simulink model "UnbalancedStarConnectedLoad1"  (Simulink 10.3)
settings: Solver=ode45  StartTime=0.0  StopTime=0.1  RelTol=1e-3  EnableMultiTasking=on
libraries: spsSeriesRLCBranchLib x5, spsACVoltageSourceLib x3, spsVoltageMeasurementLib x3, spsThreePhaseVIMeasurementLib x1, spsCurrentMeasurementLib x1, spspowerguiLib x1
settings Model: Creator=bas  LastModifiedBy=Rahul
settings DataIOCC: LimitDataPoints=on
settings DebuggingCC: SolverPrmCheckMsg=warning

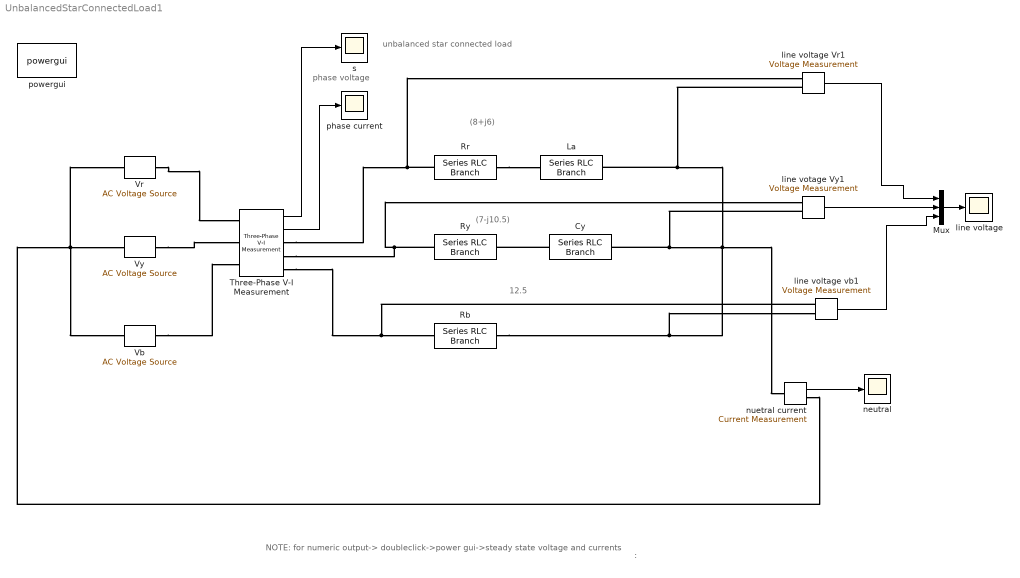
== system UnbalancedStarConnectedLoad1 ==
  note: (8+j6)
  note: (7-j10.5)
  note: 12.5
  note: :
  note: NOTE: for numeric output-> doubleclick->power gui->steady state voltage and currents
  note: unbalanced star connected load
  note: phase voltage
  " Cy" : spsSeriesRLCBranchLib/Series RLC Branch  LConnTagsString=__new0  RConnTagsString=__new0  BranchType=C  Resistance=7  Inductance=1e-3  SetiL0=off  InitialCurrent=0  Capacitance=303.15e-6  Setx0=off  InitialVoltage=0  Measurements=None
  " Ry" : spsSeriesRLCBranchLib/Series RLC Branch  LConnTagsString=__new0  RConnTagsString=__new0  BranchType=R  Resistance=7  Inductance=1e-3  SetiL0=off  InitialCurrent=0  Capacitance=1e-6  Setx0=off  InitialVoltage=0  Measurements=None
  La : spsSeriesRLCBranchLib/Series RLC Branch  LConnTagsString=__new0  RConnTagsString=__new0  BranchType=L  Resistance=15  Inductance=0.019  SetiL0=off  InitialCurrent=0  Capacitance=1e-6  Setx0=off  InitialVoltage=0  Measurements=None
  Mux : Mux  Inputs=3
  Rb : spsSeriesRLCBranchLib/Series RLC Branch  LConnTagsString=__new0  RConnTagsString=__new0  BranchType=R  Resistance=12.5  Inductance=1e-3  SetiL0=off  InitialCurrent=0  Capacitance=1e-6  Setx0=off  InitialVoltage=0  Measurements=None
  Rr : spsSeriesRLCBranchLib/Series RLC Branch  LConnTagsString=__new0  RConnTagsString=__new0  BranchType=R  Resistance=8  Inductance=1e-3  SetiL0=off  InitialCurrent=0  Capacitance=1e-6  Setx0=off  InitialVoltage=0  Measurements=None
  Three-Phase V-I Measurement : spsThreePhaseVIMeasurementLib/Three-Phase V-I Measurement  VoltageMeasurement=phase-to-phase  SetLabelV=off  LabelV=Vabc  Vpu=off  VpuLL=off  CurrentMeasurement=yes  SetLabelI=off  LabelI=Iabc  Ipu=off  Pbase=100e6  Vbase=500e3  OutputType=Complex  PhasorSimulation=off  PSBequivalent=0
  Vb : spsACVoltageSourceLib/AC Voltage Source  Amplitude=254  Phase=120  Frequency=50  SampleTime=0  Measurements=None  BusType=swing  Pref=10e3  Qref=0  Qmin=-inf  Qmax=+inf
  Vr : spsACVoltageSourceLib/AC Voltage Source  Amplitude=254  Phase=0  Frequency=50  SampleTime=0  Measurements=None  BusType=swing  Pref=10e3  Qref=0  Qmin=-inf  Qmax=+inf
  Vy : spsACVoltageSourceLib/AC Voltage Source  Amplitude=254  Phase=-120  Frequency=50  SampleTime=0  Measurements=None  BusType=swing  Pref=10e3  Qref=0  Qmin=-inf  Qmax=+inf
  line voltage : Scope
  line voltage Vr1 : spsVoltageMeasurementLib/Voltage Measurement  PhasorSimulation=off  OutputType=Complex  PSBequivalent=0
  line voltage vb1 : spsVoltageMeasurementLib/Voltage Measurement  PhasorSimulation=off  OutputType=Complex  PSBequivalent=0
  line votage Vy1 : spsVoltageMeasurementLib/Voltage Measurement  PhasorSimulation=off  OutputType=Complex  PSBequivalent=0
  neutral : Scope
  nuetral current : spsCurrentMeasurementLib/Current Measurement  PhasorSimulation=off  OutputType=Complex  PSBequivalent=0
  phase current : Scope
  powergui : spspowerguiLib/powergui  Priority=1  SimulationMode=Continuous  SampleTime=50e-6  frequency=60  Iterations=50  frequencyindice=50  Pbase=100e6  ErrMax=1e-4  UnitsV=kV  UnitsW=MW  buscounter=0  FunctionMessages=off  echomessages=off  EnableUseOfTLC=off  CurrentSourceSwitches=off  DisableSnubberDevices=off  DisableRonSwitches=off  DisableVfSwitches=off  DisplayEquations=off  AutomaticDiscreteSolvers=off  SolverType=Tustin/Backward Euler (TBE)  Interpol=off  ExternalGateDelay=off  methode=off  Ts=0  x0status=blocks  SPID=off  SwTol=0  HookPort=off  NonlinearTolerance=1e-4  nMaxIteration=100  ContinueOnMaxIteration=off  RestoreLinks=warning  ResistiveCurrentMeasurement=off  Frange=[0:2:500]  Ylog=off  Xlog=on  ShowGrid=on  save=off  variable=ZData  structure=0  ZoomFFT=off  StartTime=0.0  cycles=1  DisplayStyle=1  fundamental=60  FreqAxis=off  MaxFrequency=1000  frequencyindicesteady=1  RmsSteady=1  display=off
  s : Scope
  wires:
  line voltage Vr1/1 -> Mux/1
  line votage Vy1/1 -> Mux/2
  line voltage vb1/1 -> Mux/3
  Mux/1 -> line voltage/1
  nuetral current/1 -> neutral/1
  Three-Phase V-I Measurement/1 -> s/1
  Three-Phase V-I Measurement/2 -> phase current/1
  connections:
  " Cy"/LConn1 -- line votage Vy1/LConn2 -- nuetral current/LConn1 -- line voltage Vr1/LConn2 -- La/LConn1 -- line voltage vb1/LConn2 -- Rb/LConn1
  Rr/RConn1 -- Three-Phase V-I Measurement/RConn1 -- line voltage Vr1/LConn1
  nuetral current/RConn1 -- Vy/LConn1 -- Vr/LConn1 -- Vb/LConn1
  " Ry"/RConn1 -- line votage Vy1/LConn1 -- Three-Phase V-I Measurement/RConn2
  line voltage vb1/LConn1 -- Rb/RConn1 -- Three-Phase V-I Measurement/RConn3
  " Cy"/RConn1 -- " Ry"/LConn1
  Rr/LConn1 -- La/RConn1
  Vr/RConn1 -- Three-Phase V-I Measurement/LConn1
  Vy/RConn1 -- Three-Phase V-I Measurement/LConn2
  Vb/RConn1 -- Three-Phase V-I Measurement/LConn3
